simulink model "Slew_Following_target"  (R2026a)
settings: Solver=VariableStepAuto  StopTime=50000
values from neighbouring files (symbols this model uses):
  c = 2 * zeta * omega_n    (= 0.1)    [inizializzazione.m]
  J = [3190 0 0; 0 3790 0; 0 0 5672]    [inizializzazione.m]
  kappa = omega_n^2    (= 0.0025)    [inizializzazione.m]
  q_target = [q1; q2; q3; q4]    [inizializzazione.m]
  q_true_0 = [ -0.7125 ... (first row only)    [inizializzazione.m]
  state_0 = [q_true_0; w_true_0]    [inizializzazione.m]
  tau_m = 0.106    [inizializzazione.m]
libraries: simulink x3
settings Model: Creator=mario  LastModifiedBy=mario

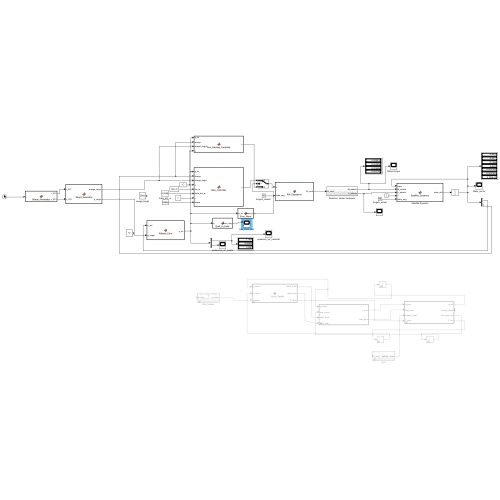
[thumbnail: Simulink's stored preview of the top-level diagram]
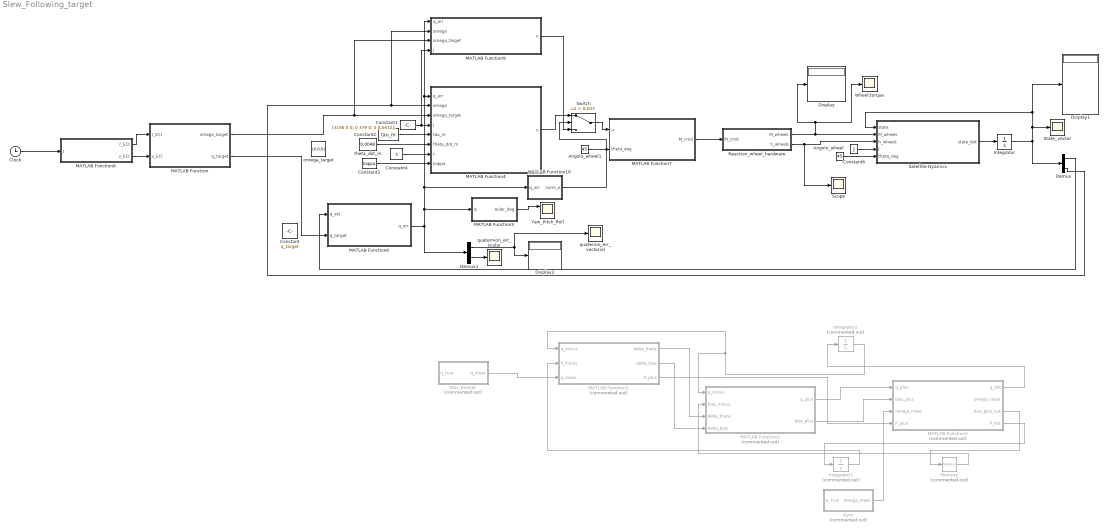
== system Slew_Following_target ==
  Angolo_wheel : Constant  Value=45
  Angolo_wheel1 : Constant  Value=45
  Clock : Clock
  Constant : Constant  Value=q_target
  Constant1 : Constant  Value=[3190 0 0; 0 379 0; 0 0 5672];
  Constant2 : Constant  Value=tau_m
  Constant3 : Constant  Value=kappa
  Constant4 : Constant  Value=c
  Constant6 : Constant  Value=J
  Demux : Demux  Outputs=2
  Demux1 : Demux  Outputs=[3 1]
  Display : Display
  Display1 : Display
  Display2 : Display
  Gyro : Subsystem  Commented=on
  Integrator : Integrator  InitialCondition=state_0
  Integrator1 : Integrator  Commented=on  InitialCondition=eye(6) * 1e-4
  Integrator2 : Integrator  Commented=on  InitialCondition=q_true_0
  MATLAB Function : MATLAB Function  TreatAsAtomicUnit=on
  MATLAB Function1 : MATLAB Function  Commented=on  TreatAsAtomicUnit=on
  MATLAB Function10 : MATLAB Function  TreatAsAtomicUnit=on
  MATLAB Function2 : MATLAB Function  Commented=on  TreatAsAtomicUnit=on
  MATLAB Function3 : MATLAB Function  Commented=on  TreatAsAtomicUnit=on
  MATLAB Function4 : MATLAB Function  TreatAsAtomicUnit=on
  MATLAB Function5 : MATLAB Function  TreatAsAtomicUnit=on
  MATLAB Function6 : MATLAB Function  TreatAsAtomicUnit=on
  MATLAB Function7 : MATLAB Function  TreatAsAtomicUnit=on
  MATLAB Function8 : MATLAB Function  TreatAsAtomicUnit=on
  MATLAB Function9 : MATLAB Function  TreatAsAtomicUnit=on
  Memory : Memory  Commented=on  InitialCondition=[0; 0; 0]
  Reaction_wheel_hardware : Subsystem
  Satellite Dyamics : MATLAB Function  TreatAsAtomicUnit=on
  Scope : Scope
      settings: DataLoggingVariableName=ScopeData5
  Star_tracker : Subsystem  Commented=on
  State_vector : Scope
      settings: ActiveDisplayYMinimum=-0.20980740065652753  ActiveDisplayYMaximum=0.16165384213934825
  Switch : Switch  Criteria=u2 > Threshold  Threshold=0.043  SaturateOnIntegerOverflow=off  InputSameDT=off
  Wheel:torque : Scope
      settings: ActiveDisplayYMinimum=-0.072655763047117392  ActiveDisplayYMaximum=0.050852529352741559
  Yaw_Pitch_Roll : Scope  NumInputPorts=2
      settings: ActiveDisplayYMinimum=-199.32266447947097  ActiveDisplayYMaximum=199.34044920108022  DataLoggingVariableName=ScopeData2
  omega_target : Constant  Value=[0;0;0]
  quaterion_err_vectorial : Scope
      settings: ActiveDisplayYMinimum=-1.4884542786746136  ActiveDisplayYMaximum=1.6627998642060726  DataLoggingVariableName=ScopeData3
  quaternion_err_scalar : Scope
      settings: ActiveDisplayYMinimum=-0.87381284022924977  ActiveDisplayYMaximum=1.9707894578453811  DataLoggingVariableName=ScopeData4
  theta_dot_m : Constant  Value=0.0048
  wires:
  Reaction_wheel_hardware/2(h_wheels) -> Scope/1, Satellite Dyamics/3(h_wheels)
  Satellite Dyamics/1(state_dot) -> Integrator/1
  MATLAB Function1/1(delta_theta) -> MATLAB Function2/3(delta_theta)
  MATLAB Function1/2(delta_bias) -> MATLAB Function2/4(delta_bias)
  MATLAB Function2/1(q_plus) -> MATLAB Function3/1(q_plus)
  MATLAB Function2/2(bias_plus) -> MATLAB Function3/2(bias_plus)
  theta_dot_m/1 -> MATLAB Function4/6(theta_dot_m)
  MATLAB Function3/1(q_dot) -> Integrator2/1
  Integrator2/1 -> MATLAB Function2/1(q_minus), MATLAB Function1/1(q_minus)
  MATLAB Function3/4(P_dot) -> Integrator1/1
  Integrator1/1 -> MATLAB Function1/2(P_minus)
  Star_tracker/1(q_meas) -> MATLAB Function1/3(q_meas)
  Gyro/1(omega_meas) -> MATLAB Function3/3(omega_meas)
  MATLAB Function1/3(P_plus) -> MATLAB Function3/4(P_plus)
  MATLAB Function3/3(bias_plus_out) -> Memory/1
  Memory/1 -> MATLAB Function2/2(bias_minus)
  Demux/2 -> MATLAB Function9/2(omega), MATLAB Function4/2(omega)
  Demux/1 -> MATLAB Function6/1(q_est)
  Constant4/1 -> MATLAB Function4/7(c)
  Constant3/1 -> MATLAB Function4/8(kappa)
  Constant2/1 -> MATLAB Function4/5(tau_m)
  MATLAB Function5/1(euler_deg) -> Yaw_Pitch_Roll/1
  Demux1/2 -> quaternion_err_scalar/1
  Constant1/1 -> MATLAB Function9/4(J), MATLAB Function4/4(J)
  Constant6/1 -> Satellite Dyamics/4(J)
  MATLAB Function7/1(M_cmd) -> Reaction_wheel_hardware/1(M_cmd)
  Reaction_wheel_hardware/1(M_wheels) -> Display/1, Wheel:torque/1, Satellite Dyamics/2(M_wheels)
  Angolo_wheel/1 -> Satellite Dyamics/5(theta_deg)
  Angolo_wheel1/1 -> MATLAB Function7/2(theta_deg)
  MATLAB Function6/1(q_err) -> MATLAB Function10/1(q_err), MATLAB Function9/1(q_err), MATLAB Function4/1(q_err), MATLAB Function5/1(q), Demux1/1
  Demux1/1 -> Display2/1, quaterion_err_vectorial/1
  Integrator/1 -> Demux/1, State_vector/1, Display1/1, Satellite Dyamics/1(state)
  Clock/1 -> MATLAB Function8/1(t)
  MATLAB Function8/2(v_ECI) -> MATLAB Function/2(v_ECI)
  MATLAB Function8/1(r_ECI) -> MATLAB Function/1(r_ECI)
  MATLAB Function/1(omega_target) -> MATLAB Function9/3(omega_target), MATLAB Function4/3(omega_target)
  MATLAB Function/2(q_target) -> MATLAB Function6/2(q_target)
  MATLAB Function4/1(u) -> Switch/1
  MATLAB Function9/1(u) -> Switch/3
  Switch/1 -> MATLAB Function7/1(u)
  ? -> ?
  MATLAB Function10/1(norm_e) -> Switch/2

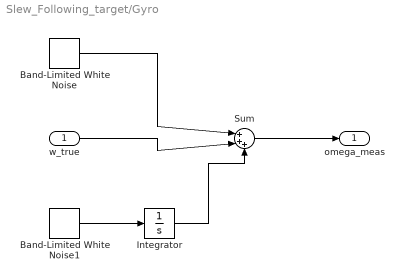
== system Slew_Following_target/Gyro ==
  w_true : Inport
  Band-Limited White Noise : simulink/Sources/Band-Limited White Noise  Cov=[1e-6; 1e-6; 1e-6]  Ts=0.1  seed=[1; 2; 3]
  Band-Limited White Noise1 : simulink/Sources/Band-Limited White Noise  Cov=[1e-6; 1e-6; 1e-6]  Ts=0.1  seed=[5; 6; 7]
  Integrator : Integrator
  Sum : Sum  Inputs=|+++
  omega_meas : Outport
  wires:
  Band-Limited White Noise1/1 -> Integrator/1
  Integrator/1 -> Sum/3
  w_true/1 -> Sum/2
  Band-Limited White Noise/1 -> Sum/1
  Sum/1 -> omega_meas/1

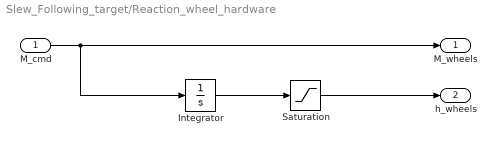
== system Slew_Following_target/Reaction_wheel_hardware ==
  M_cmd : Inport  PortDimensions=4
  Integrator : Integrator  InitialCondition=[0; 0; 0; 0]  LimitOutput=on  UpperSaturationLimit=12  LowerSaturationLimit=-12
  Saturation : Saturate  UpperLimit=50  LowerLimit=-50
  M_wheels : Outport
  h_wheels : Outport  Port=2
  wires:
  M_cmd/1 -> Integrator/1, M_wheels/1
  Integrator/1 -> Saturation/1
  Saturation/1 -> h_wheels/1

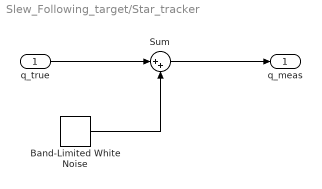
== system Slew_Following_target/Star_tracker ==
  q_true : Inport
  Band-Limited White Noise : simulink/Sources/Band-Limited White Noise  Cov=[1e-5; 1e-5; 1e-5; 1e-5]  Ts=0.1  seed=[1; 2; 3; 4]
  Sum : Sum  Inputs=|++
  q_meas : Outport
  wires:
  q_true/1 -> Sum/1
  Band-Limited White Noise/1 -> Sum/2
  Sum/1 -> q_meas/1

== matlab function Slew_Following_target/MATLAB Function8 ==
  data: t input; r_ECI output; v_ECI output
function [r_ECI, v_ECI] = Orbital_Kinematics(t)
    % 1. PARAMETRI ORBITALI (Devono coincidere con quelli di inizializzazione)
    mu = 3.986e14;          
    R_E = 6378.1363e3;      
    alt = 600e3;            
    a = R_E + alt;          
    
    % Inclinazione, RAAN e anomalia iniziale (convertiti in rad)
    inc = 98 * (pi/180);    
    RAAN = 0;               % Se hai RAAN = 0 nel workspace, usa 0
    om = 0;                 % Anomalia/Argomento iniziale
    
    % Rateo orbitale costante
    omega_orb = sqrt(mu / a^3);
    
    % 2. CALCOLO ANGOLO ISTANTANEO (Argomento di latitudine)
    theta = omega_orb * t + om;
    
    % 3. VETTORE POSIZIONE r_ECI [m]
    r_ECI = zeros(3,1);
    r_ECI(1) = a * (cos(RAAN)*cos(theta) - sin(RAAN)*sin(theta)*cos(inc));
    r_ECI(2) = a * (sin(RAAN)*cos(theta) + cos(RAAN)*sin(theta)*cos(inc));
    r_ECI(3) = a * sin(inc)*sin(theta);
    
    % 4. VETTORE VELOCITÀ v_ECI [m/s] (Derivata analitica di r_ECI)
    v_ECI = zeros(3,1);
    v_ECI(1) = a * omega_orb * (-cos(RAAN)*sin(theta) - sin(RAAN)*cos(theta)*cos(inc));
    v_ECI(2) = a * omega_orb * (-sin(RAAN)*sin(theta) + cos(RAAN)*cos(theta)*cos(inc));
    v_ECI(3) = a * omega_orb * (sin(inc)*cos(theta));
end

== matlab function Slew_Following_target/MATLAB Function9 ==
  data: q_err input; u output; omega input; omega_target input; J input
function u  = Fine_Pointing_Controller(q_err, omega, omega_target, J)
    % 1. ESTRAZIONE STATO (Ipotesi piccoli angoli)
    
    qe1 = q_err(1); qe2 = q_err(2); qe3 = q_err(3); qe4 = q_err(4);
    R_LVLH_to_Body = [qe4^2+qe1^2-qe2^2-qe3^2,   2*(qe1*qe2+qe4*qe3),       2*(qe1*qe3-qe4*qe2);
        2*(qe1*qe2-qe4*qe3),       qe4^2-qe1^2+qe2^2-qe3^2,   2*(qe2*qe3+qe4*qe1);
        2*(qe1*qe3+qe4*qe2),       2*(qe2*qe3-qe4*qe1),       qe4^2-qe1^2-qe2^2+qe3^2];

    omega_target_body = R_LVLH_to_Body * omega_target;
    delta_omega = omega - omega_target_body;

    q_vec = q_err(1:3);
    delta_omega = omega - omega_target;

    % 2. TUNING LINEARE (Fine Pointing)
    % Impostiamo una frequenza naturale molto dolce (wn) e smorzamento critico (zeta)
    % per un inseguimento fluido che non stressi le ruote di reazione.
    wn = 0.01;      % Frequenza di circa 0.01 rad/s (lenta e morbida)
    zeta = 1.0;     % Smorzamento critico (nessuna oscillazione)

    Kp = (wn^2) * J;                % Matrice "Molla" proporzionale
    Kd = (2 * zeta * wn) * J;       % Matrice "Freno" derivativo

    % 3. LEGGE DI CONTROLLO PD LINEARE PER TRACKING
    tau_req = Kp * q_vec + Kd * delta_omega;

    % 4. SATURAZIONE DI SICUREZZA E COMANDO MOTORI
    tau_m = 0.075; % Limite Collins
    sigma = max(abs(tau_req) / tau_m);
    
    if sigma > 1
        u = -tau_req / sigma;  % Preserva la direzione vettoriale
    else
        u = -tau_req;
    end
end

== matlab function Slew_Following_target/MATLAB Function10 ==
  data: q_err input; norm_e output
function norm_e = Error_Norm(q_err)
    % Questa funzione riceve il quaternione 4x1, 
    % estrae i primi 3 elementi e ne calcola la grandezza scalare.
    
    q_vec = q_err(1:3);      % Estrae la parte vettoriale
    norm_e = norm(q_vec);    % Calcola la norma pitagorica (Singolo numero)
end

== matlab function Slew_Following_target/MATLAB Function1 ==
  data: q_minus input size=[4 1]; delta_theta output size=[3 1]; P_minus input size=[6 6 ]; q_meas input size=[4 1]; delta_bias output size=[3 1]; P_plus output size=[6 6]
function [delta_theta, delta_bias, P_plus] = MEKF_Error_Update(q_minus, P_minus, q_meas)
    % 1. MODELLO DI MISURA
    H = [eye(3), zeros(3,3)]; 
    sigma_ST = (10 / 3600) * (pi / 180); % Rumore Star Tracker (es. 10 arcosecondi)
    R = (sigma_ST^2) * eye(3);

    % 2. CALCOLO DELL'INNOVAZIONE (Errore di Quaternione)
    q_inv = [-q_minus(1:3); q_minus(4)];
    % Moltiplicazione q_meas (X) q_minus^(-1)
    delta_q_meas = [q_inv(4)*q_meas(1:3) + q_meas(4)*q_inv(1:3) - cross(q_meas(1:3), q_inv(1:3));
                    q_meas(4)*q_inv(4) - dot(q_meas(1:3), q_inv(1:3))];
    
    if delta_q_meas(4) < 0
        delta_q_meas = -delta_q_meas; % Forziamo rotazione minima
    end
    y_k = 2 * delta_q_meas(1:3); % Vettore di errore (Rodrigues approssimato)

    % 3. GUADAGNO DI KALMAN
    S = H * P_minus * H' + R;
    K = P_minus * H' / S;

    % 4. AGGIORNAMENTO DELLO STATO DI ERRORE
    delta_x_plus = K * y_k;
    delta_theta = delta_x_plus(1:3);
    delta_bias  = delta_x_plus(4:6);

    % 5. AGGIORNAMENTO COVARIANZA
    P_plus = (eye(6) - K * H) * P_minus;
    P_plus = 0.5 * (P_plus + P_plus'); % Forza simmetria matematica
end

== matlab function Slew_Following_target/Satellite Dyamics ==
  data: state input; state_dot output; M_wheels input; h_wheels input; J input; theta_deg input
function state_dot = Satellite_Dynamics(state, M_wheels, h_wheels, J, theta_deg)

    %% 0. MESSA IN SICUREZZA DELLE DIMENSIONI (Evita gli errori di compilazione Simulink)
    % Dichiariamo subito la dimensione dell'uscita
    state_dot = zeros(7,1); 
    
    % Forziamo tutti i segnali in ingresso a essere vettori colonna (Nx1)
    state = state(:);
    M_wheels = M_wheels(:);
    h_wheels = h_wheels(:);
    
    % Assicuriamoci che l'angolo sia uno scalare
    theta_deg = theta_deg(1);

    %% 1. ESTRAZIONE DELLO STATO
    % Quaternione (Convenzione Scalar-Last)
    q = state(1:4); 
    % Velocità angolare [rad/s]
    w = state(5:7); 

    %% 2. MATRICE DELLA GEOMETRIA DELLE RUOTE
    theta = theta_deg * (pi/180); 
    
    % Matrice di attuazione Aw per la configurazione a 4 ruote inclinate
    Aw = [ cos(theta),      0,       -cos(theta),      0;
           sin(theta),  sin(theta),   sin(theta),  sin(theta);
               0,      -cos(theta),       0,       cos(theta)];
               
    % Proiezione dai 4 assi delle ruote ai 3 assi del corpo
    M_contr = Aw * M_wheels; 
    h_w_contr = Aw * h_wheels; 

    %% 3. DINAMICA ROTAZIONALE (Equazioni di Eulero Accoppiate)
    skew_w = [   0,   -w(3),   w(2);
               w(3),     0,  -w(1);
              -w(2),   w(1),     0 ];
              % bigogna inserire il contributo di gravity gradient e
              % external torque nella formula sotto
              
    w_dot = J \ (-M_contr - skew_w * (J * w + h_w_contr)); 

    %% 4. CINEMATICA D'ASSETTO (Derivata del Quaternione)
    q_v = q(1:3); 
    q_s = q(4);   
    
    q_v_dot = -0.5 * skew_w * q_v + 0.5 * q_s * w;
    q_s_dot = -0.5 * w' * q_v;
    
    q_dot = [q_v_dot; q_s_dot];

    %% 5. ASSEMBLAGGIO DELL'USCITA
    state_dot = [q_dot; w_dot];
    % Calcolo dell'errore di norma del quaternione
    norm_err = 1 - (q(1)^2 + q(2)^2 + q(3)^2 + q(4)^2);
    k_norm = 0.05; % Abbassato da 10 per garantire stabilità numerica

    % Aggiungiamo il termine di Baumgarte alla derivata
    q_dot = [q_v_dot; q_s_dot] + k_norm * norm_err * q;

    % Vettore di stato derivato in uscita
    state_dot = [q_dot; w_dot];
end

== matlab function Slew_Following_target/MATLAB Function2 ==
  data: q_minus input; q_plus output; bias_plus output; bias_minus input; delta_theta input; delta_bias input
function [q_plus, bias_plus] = MEKF_Reset(q_minus, bias_minus, delta_theta, delta_bias)
    % 1. AGGIORNAMENTO DEL BIAS
    bias_plus = bias_minus + delta_bias;

    % 2. AGGIORNAMENTO DEL QUATERNIONE (Moltiplicativo)
    q_err = [delta_theta / 2; 1];
    q_tmp = [q_minus(4)*q_err(1:3) + q_err(4)*q_minus(1:3) - cross(q_err(1:3), q_minus(1:3));
             q_err(4)*q_minus(4) - dot(q_err(1:3), q_minus(1:3))];

    % Normalizzazione Brute Force
    q_plus = q_tmp / norm(q_tmp);
end

== matlab function Slew_Following_target/MATLAB Function3 ==
  data: q_plus input; q_dot output; bias_plus input; omega_meas input; omega_clean output; bias_plus_out output; P_plus input; P_dot output
function [q_dot, omega_clean, bias_plus_out, P_dot] = MEKF_Propagation(q_plus, bias_plus, omega_meas, P_plus)
    bias_plus_out = bias_plus; % Il bias si stima costante nella propagazione

    % 1. VELOCITÀ ANGOLARE DEPURATA DAL BIAS
    omega_clean = omega_meas - bias_plus;

    % 2. CINEMATICA DEL QUATERNIONE
    w = omega_clean;
    skew_w = [   0,  -w(3),   w(2);
               w(3),     0,  -w(1);
              -w(2),  w(1),     0 ];
              
    q_v = q_plus(1:3); q_s = q_plus(4);
    q_v_dot = -0.5 * skew_w * q_v + 0.5 * q_s * w;
    q_s_dot = -0.5 * w' * q_v;
    q_dot = [q_v_dot; q_s_dot];

    % 3. PROPAGAZIONE DELLA COVARIANZA (Aggiunta Fondamentale)
    % Matrice della Dinamica F [6x6]
    F = [ -skew_w,  -eye(3);
          zeros(3,3), zeros(3,3) ];
          
    % Matrice Rumore di Processo Q [6x6]
    sigma_v = sqrt(10) * 1e-6; % ARW dei giroscopi
    sigma_u = sqrt(10) * 1e-9; % RRW (instabilità del bias)
    Q = blkdiag((sigma_v^2)*eye(3), (sigma_u^2)*eye(3));

    % Derivata di Riccati
    P_dot = F * P_plus + P_plus * F' + Q;
end

== matlab function Slew_Following_target/MATLAB Function4 ==
  data: q_err input; u output; omega input; omega_target input; J input; tau_m input; theta_dot_m input; c input; kappa input
function u = Slew_Controller(q_err, omega, omega_target, J, tau_m, theta_dot_m, c, kappa)
    % 1. ESTRAZIONE E COSTRUZIONE MATRICE (Da LVLH a Body)
 
    q_vec = q_err(1:3);
    qe1 = q_err(1); qe2 = q_err(2); qe3 = q_err(3); qe4 = q_err(4);
    
    R_LVLH_to_Body = [qe4^2+qe1^2-qe2^2-qe3^2,   2*(qe1*qe2+qe4*qe3),       2*(qe1*qe3-qe4*qe2);
        2*(qe1*qe2-qe4*qe3),       qe4^2-qe1^2+qe2^2-qe3^2,   2*(qe2*qe3+qe4*qe1);
        2*(qe1*qe3+qe4*qe2),       2*(qe2*qe3-qe4*qe1),       qe4^2-qe1^2-qe2^2+qe3^2];
    
    % Proietto la velocità del target nel sistema di riferimento del satellite
    omega_target_body = R_LVLH_to_Body * omega_target;
    
    % 2. ERRORE DI VELOCITA' (Ora la sottrazione è fisicamente coerente)
    delta_omega = omega - omega_target_body;

    % 1. ERRORE DI ASSETTO E DI VELOCITÀ RELATIVA
    q_e = q_err(1:3);
    norm_qe = norm(q_e);

    % La velocità relativa al bersaglio orbitale (Inseguimento)
    % delta_omega = omega - omega_target;

    % Sicurezza: se l'errore è microscopico, spegni i motori e risparmia energia
    if norm_qe < 1e-6
        u = [0; 0; 0];
        return;
    end

    % 2. CALCOLO DEI GUADAGNI DEL CONTROLLORE DI KJELLBERG
    % C è il "freno" (Azione derivativa)
    C = c * J;

    % K è la "molla" proporzionale per ogni asse
    k1 = c * (abs(q_e(1)) / norm_qe) * theta_dot_m;
    k2 = c * (abs(q_e(2)) / norm_qe) * theta_dot_m;
    k3 = c * (abs(q_e(3)) / norm_qe) * theta_dot_m;
    K = diag([k1, k2, k3]) * J;

    % 3. CALCOLO DELLA VELOCITÀ DESIDERATA (Senza divisioni per zero)
    % Uso 'epsilon' per evitare che il calcolo esploda e per addolcire la frenata
    epsilon = 0.043; 
    coeff = (kappa * norm_qe) / (c * theta_dot_m);
    
    v_in = zeros(3,1);
    v_in(1) = coeff * (q_e(1) / (abs(q_e(1)) + epsilon));
    v_in(2) = coeff * (q_e(2) / (abs(q_e(2)) + epsilon));
    v_in(3) = coeff * (q_e(3) / (abs(q_e(3)) + epsilon));

    % 4. SATURAZIONE INTERNA
    % Taglia la richiesta matematica se l'errore iniziale di 140° è troppo grande
    v_sat = max(min(v_in, 1), -1);

    % 5. COPPIA TEORICA (Molla proporzionale + Freno derivativo)
    tau = K * v_sat + C * delta_omega;

    % 6. SATURAZIONE ESTERNA HARDWARE
    % Se la coppia calcolata supera i limiti fisici delle ruote, la riduce
    % in proporzione per non perdere la direzione della manovra di Slew
    sigma = max(abs(tau) / tau_m);
    if sigma > 1
        u = -tau / sigma;
    else
        u = -tau;
    end
end

== matlab function Slew_Following_target/MATLAB Function5 ==
  data: q input; euler_deg output
function euler_deg = Quat_to_Euler(q)
% INGRESSO: q (Quaternione 4x1, convenzione Scalar-Last)
% USCITA: euler_deg (Vettore 3x1 con [Roll; Pitch; Yaw] in GRADI)

% 1. Estrazione degli elementi del quaternione
q1 = q(1);
q2 = q(2);
q3 = q(3);
q4 = q(4); % Elemento scalare

% 2. Calcolo dei soli elementi della Matrice di Rotazione (DCM) necessari
% Formule basate sulla trasformazione Quaternione -> DCM
M11 = q1^2 - q2^2 - q3^2 + q4^2;
M12 = 2 * (q1*q2 + q3*q4);
M13 = 2 * (q1*q3 - q2*q4);
M23 = 2 * (q2*q3 + q1*q4);
M33 = -q1^2 - q2^2 + q3^2 + q4^2;

% 3. Estrazione degli angoli di Eulero (Sequenza 3-2-1)

% ROLLIO (Roll / Phi) - Rotazione attorno asse X
roll = atan2(M23, M33);

% BECCHEGGIO (Pitch / Theta) - Rotazione attorno asse Y
% Aggiungiamo una protezione numerica per evitare che errori di
% arrotondamento portino l'argomento di asin fuori da [-1, 1],
% il che genererebbe numeri complessi e manderebbe in blocco Simulink.
sin_p = -M13;
sin_p = max(min(sin_p, 1), -1);
pitch = asin(sin_p);

% IMBARDATA (Yaw / Psi) - Rotazione attorno asse Z
yaw = atan2(M12, M11);

% 4. Conversione in GRADI e assemblaggio del vettore in uscita
euler_deg = [roll; pitch; yaw] * (180 / pi);
end

== matlab function Slew_Following_target/MATLAB Function6 ==
  data: q_est input size=[4 1]; q_err output size=[4 1]; q_target input size=[4 1]
function q_err = Attitude_Error(q_est, q_target)
    % 1. Calcola l'inverso del quaternione target (Convenzione Scalar-Last)
    % L'inverso di un quaternione unitario coincide con il suo coniugato
    q_target_inv = [-q_target(1:3); q_target(4)];
    
    % 2. Moltiplicazione quaternionica: q_target_inv (X) q_est
    % Applichiamo rigorosamente la formula del prodotto per la convenzione Scalar-Last
    q_err_vec = q_est(4)*q_target_inv(1:3) + q_target_inv(4)*q_est(1:3) - cross(q_est(1:3), q_target_inv(1:3));
    q_err_sca = q_target_inv(4)*q_est(4) - dot(q_target_inv(1:3), q_est(1:3));
    
    q_err = [q_err_vec; q_err_sca];
    
    % 3. Forziamo la rotazione minima (Shortest path)
    % Evita che il satellite compia una rotazione maggiore di 180 gradi
    if q_err(4) < 0
        q_err = -q_err;
    end
end

== matlab function Slew_Following_target/MATLAB Function7 ==
  data: u input; M_cmd output; theta_deg input
function M_cmd = RW_Dispatcher(u, theta_deg)
    % u: Coppia desiderata sui 3 assi del satellite (dal Slew_Controller)
    % theta: angolo di inclinazione delle ruote (es. 45 * pi/180)
    theta = theta_deg * (pi/180); 
    % Matrice di configurazione hardware a 4 ruote inclinate
    Aw = [cos(theta),          0, -cos(theta),           0;
          sin(theta), sin(theta),  sin(theta),  sin(theta);
                   0, -cos(theta),          0,  cos(theta)];
          
    % Calcolo della Right Pseudoinverse
    Aw_pinv = pinv(Aw);
    
    % Distribuzione della coppia: minimizza l'energia spesa dalle 4 ruote
    M_cmd = Aw_pinv * (-u);
end

== matlab function Slew_Following_target/MATLAB Function ==
  data: omega_target output; r_ECI input; q_target output; v_ECI input
function [omega_target,q_target] = Target_Generator(r_ECI, v_ECI)
    
    % 1. Calcolo dinamico degli assi LVLH in coordinate ECI
    % L'asse Z (Nadir) punta verso il centro della Terra
    z_o = -r_ECI / norm(r_ECI); 
    
    % L'asse Y (Normale all'orbita) è opposto al momento angolare
    h_orb = cross(r_ECI, v_ECI);
    y_o = -h_orb / norm(h_orb); 
    
    % L'asse X completa la terna destrorsa (direzione del moto)
    x_o = cross(y_o, z_o); 
    
    % 2. Costruzione della matrice di rotazione istantanea (Da ECI a LVLH)
    A_IO = [x_o, y_o, z_o]; % Matrice da LVLH a ECI
    A_OI = A_IO';           % Matrice da ECI a LVLH (Target)
    
    % 3. Conversione in Quaternione (Scalar-Last) in tempo reale
    tr = trace(A_OI);
    q4 = 0.5 * sqrt(1 + tr);
    q1 = (A_OI(2,3) - A_OI(3,2)) / (4*q4);
    q2 = (A_OI(3,1) - A_OI(1,3)) / (4*q4);
    q3 = (A_OI(1,2) - A_OI(2,1)) / (4*q4);
    
    q_target = [q1; q2; q3; q4];
    
    % 4. Calcolo della Velocità Angolare del Bersaglio
    % In un'orbita circolare, l'LVLH ruota attorno all'asse Y (negativo) 
    % con un rateo pari al rateo orbitale omega_0.
    omega_0 = norm(h_orb) / (norm(r_ECI)^2); 
    omega_target = [0; -omega_0; 0];
    
end
